simulink model "Heli_Simulation_VR1"  (R2024b)
settings: Solver=FixedStepAuto  StartTime=0.0  StopTime=50  RelTol=1e-3  EnableMultiTasking=on
values from neighbouring files (symbols this model uses):
  D2R = pi/180.0    (= 0.0174532925199)    [Heli_Setup.m]
  ELEV_SLF = 24.25    [Heli_Setup.m]
  ELEV_START = -24.25    [Heli_Setup.m]
  Kd = 128    [Heli_Setup.m]
  Kdt = 1.38e3    (= 1380)    [Heli_Setup.m]
  Ki = 63.5    [Heli_Setup.m]
  Kit = 43.4    [Heli_Setup.m]
  Kp = 84.1    [Heli_Setup.m]
  Kpt = 448    [Heli_Setup.m]
  R2D = 180/pi    (= 57.2957795131)    [Heli_Setup.m]
  VSUM_MAX = 36    [Heli_Setup.m]
undefined symbols (not defined in the file or in its folder): YAW_SP, YAW_START
libraries: vrlib x7, cstblocks x2
Description:
  | Simulink(R) 3D Animation(TM) - Tutorial #3
  | 
  | Tutorial model to be used for 3D World Editor authoring example in the documentation.
  | After creating the virtual world according to the instructions in the documentation, include the VR block
  | in the model and connect B1, B2 coordinates and S scaling to corresponding nodes in
  | the virtual world.
settings Model: Creator=Danek  LastModifiedBy=bryankikuta
settings SolverCC: ConcurrentTasks=on  AlgebraicLoopSolver=TrustRegion  AutoInsertRateTranBlk=on  InsertRTBMode=Never (minimum delay)
settings DataIOCC: LimitDataPoints=on  SaveFormat=StructureWithTime  SignalLoggingSaveFormat=ModelDataLogs  SaveOutput=off  SaveTime=off  ReturnWorkspaceOutputs=off  SignalLoggingName=logsOut
settings OptimizationCC: BlockReduction=off  BooleanDataType=off  DefaultParameterBehavior=Inlined  OptimizeBlockIOStorage=off  BufferReuse=off  GlobalBufferReuse=off  ExpressionFolding=off  PassReuseOutputArgsThreshold=0  ExpressionDepthLimit=2147483647  LocalBlockOutputs=off  InitFltsAndDblsToZero=on
settings DebuggingCC: UnderspecifiedInitializationDetection=Classic  MergeDetectMultiDrivingBlocksExec=none  CheckExecutionContextPreStartOutputMsg=on  SignalResolutionControl=TryResolveAllWithWarning  ParameterTunabilityLossMsg=error  FcnCallInpInsideContextMsg=warning  UnconnectedInputMsg=warning  UnconnectedOutputMsg=warning  UnconnectedLineMsg=warning  StateNameClashWarn=warning  SFUnexpectedBacktrackingDiag=warning  SFNoUnconditionalDefaultTransitionDiag=warning  SFExecutionAtInitializationDiag=none  ArithmeticOperatorsInVariantConditions=warning
settings HardwareCC: TargetBitPerLong=64  TargetBitPerPointer=64  TargetBitPerSizeT=64  TargetBitPerPtrDiffT=64  TargetLongLongMode=on  TargetIntDivRoundTo=Zero  TargetEndianess=LittleEndian  TargetWordSize=64  TargetHWDeviceType=MATLAB Host
settings ModelReferenceCC: UpdateModelReferenceTargets=IfOutOfDate  EnableRefExpFcnMdlSchedulingChecks=on  PropagateSignalLabelsOutOfModel=off
settings SFSimCC: SimUseLocalCustomCode=off  MATLABDynamicMemAlloc=off  CustomCodeUndefinedFunction=UseInterfaceOnly
settings RTWCC: GenerateReport=on  RTWUseLocalCustomCode=off  LaunchReport=on  RTWCompilerOptimization=on  GPUComputeCapability=3.5
settings CodeAppCC: ForceParamTrailComments=on  MaxIdLength=95  OperatorAnnotations=on  StateflowObjectComments=on  MATLABSourceComments=on
settings GRTTargetCC: TargetLangStandard=C89/C90 (ANSI)
settings ConfigComp: CovMetricSettings=d  CovSaveCumulativeToWorkspaceVar=on  CovSaveSingleToWorkspaceVar=on  CovExternalEMLEnable=off

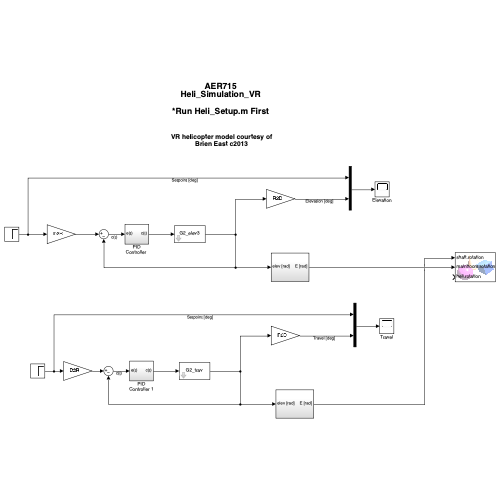
[thumbnail: Simulink's stored preview of the top-level diagram]
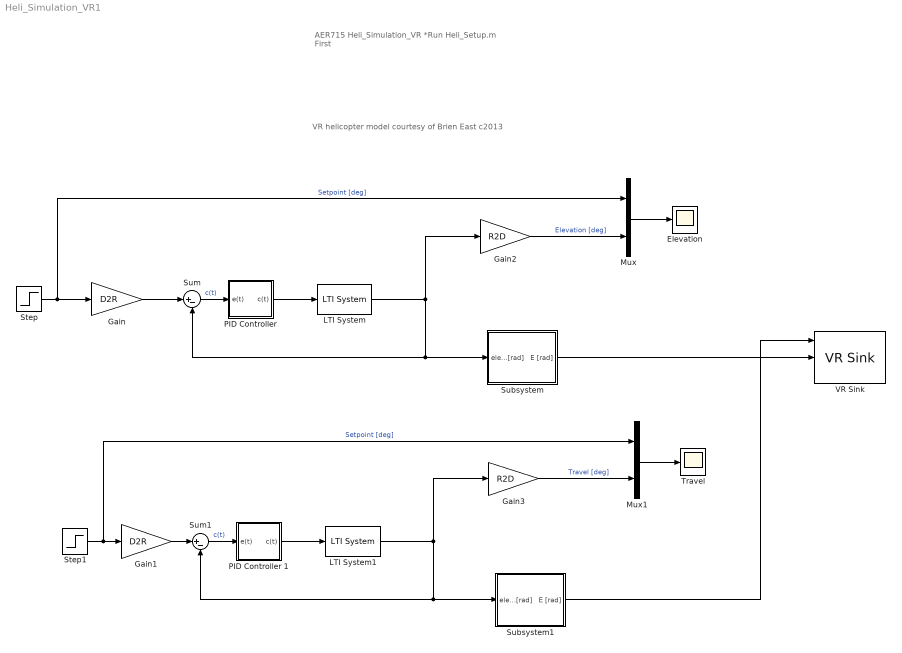
== system Heli_Simulation_VR1 ==
  note: AER715
      | Heli_Simulation_VR
      |
      | *Run Heli_Setup.m First
  note: VR helicopter model courtesy of
      | Brien East c2013
  " PID Controller " : Subsystem
  " PID Controller 1" : Subsystem
  Elevation : Scope
  Gain : Gain  Gain=D2R
  Gain1 : Gain  Gain=D2R
  Gain2 : Gain  Gain=R2D
  Gain3 : Gain  Gain=R2D
  LTI System : cstblocks/LTI System  sys=G2_elev3  IC=[]  PadeOrder=0
  LTI System1 : cstblocks/LTI System  sys=G2_trav  IC=[]  PadeOrder=0
  Mux : Mux  Inputs=2
  Mux1 : Mux  Inputs=2
  Step : Step  Before=ELEV_START  After=ELEV_SLF  SampleTime=0.1
  Step1 : Step  Before=YAW_START  After=YAW_SP  SampleTime=0.1
  Subsystem : Subsystem
  Subsystem1 : Subsystem
  Sum : Sum  Inputs=|+-
  Sum1 : Sum  Inputs=|+-
  Travel : Scope
  VR Sink : vrlib/VR Sink  InstantiateOnLoad=on  SampleTime=-1  ViewEnable=on  RemoteChange=off  RemoteView=off  FieldsWritten=shaft.rotation.4.1.1.double#mainboom.rotation.4.1.1.double#heli.rotation.4.1.1.double  WorldFileName=heliMain.wrl  AutoView=on  VideoDimensions=[]  AllowVariableSize=off
  wires:
  LTI System/1 -> Gain2/1, Sum/2, Subsystem/1(elev [rad])
  Subsystem/1(E [rad]) -> VR Sink/2
  Gain/1 -> Sum/1
  Sum/1 -> " PID Controller "/1(e(t))  "c(t)"
  " PID Controller "/1(c(t)) -> LTI System/1
  Gain2/1 -> Mux/2  "Elevation [deg]"
  Mux/1 -> Elevation/1
  Step/1 -> Gain/1, Mux/1  "Setpoint [deg]"
  LTI System1/1 -> Gain3/1, Sum1/2, Subsystem1/1(elev [rad])
  Subsystem1/1(E [rad]) -> VR Sink/1
  Gain1/1 -> Sum1/1
  Sum1/1 -> " PID Controller 1"/1(e(t))  "c(t)"
  " PID Controller 1"/1(c(t)) -> LTI System1/1
  Gain3/1 -> Mux1/2  "Travel [deg]"
  Mux1/1 -> Travel/1
  Step1/1 -> Gain1/1, Mux1/1  "Setpoint [deg]"

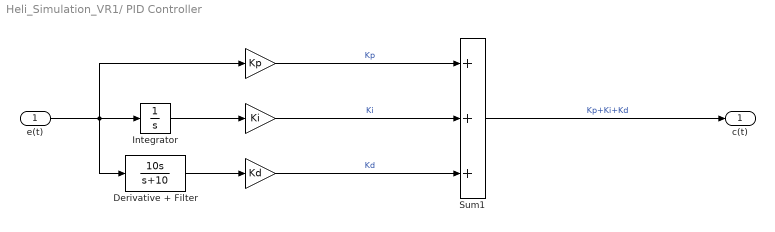
== system Heli_Simulation_VR1/ PID Controller  ==
  e(t) : Inport
  " " : Gain  Gain=Kp
  "  " : Gain  Gain=Ki
  "   " : Gain  Gain=Kd
  Derivative + Filter : TransferFcn  Numerator=[10 0]  Denominator=[1 10]
  Integrator : Integrator  UpperSaturationLimit=30  LowerSaturationLimit=-30
  Sum1 : Sum  Inputs=+++
  c(t) : Outport
  wires:
  " "/1 -> Sum1/1  "Kp"
  Sum1/1 -> c(t)/1  "Kp+Ki+Kd"
  "  "/1 -> Sum1/2  "Ki"
  "   "/1 -> Sum1/3  "Kd"
  Derivative + Filter/1 -> "   "/1
  Integrator/1 -> "  "/1
  e(t)/1 -> Integrator/1, Derivative + Filter/1, " "/1

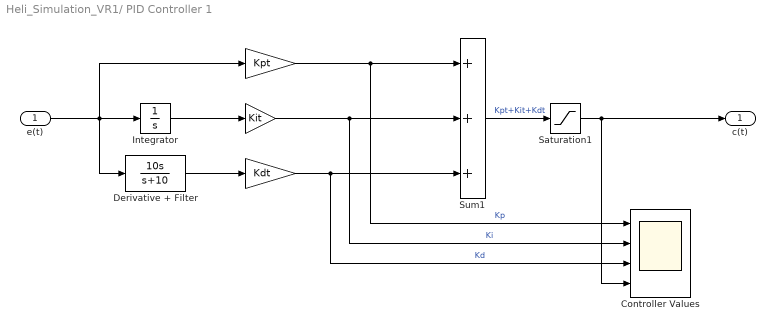
== system Heli_Simulation_VR1/ PID Controller 1 ==
  e(t) : Inport
  " " : Gain  Gain=Kpt
  "  " : Gain  Gain=Kit
  "   " : Gain  Gain=Kdt
  Controller Values : Scope  NumInputPorts=4
  Derivative + Filter : TransferFcn  Numerator=[10 0]  Denominator=[1 10]
  Integrator : Integrator  UpperSaturationLimit=30  LowerSaturationLimit=-30
  Saturation1 : Saturate  UpperLimit=VSUM_MAX  LowerLimit=-VSUM_MAX
  Sum1 : Sum  Inputs=+++
  c(t) : Outport
  wires:
  " "/1 -> Sum1/1, Controller Values/1  "Kp"
  "  "/1 -> Sum1/2, Controller Values/2  "Ki"
  "   "/1 -> Sum1/3, Controller Values/3  "Kd"
  Derivative + Filter/1 -> "   "/1
  Integrator/1 -> "  "/1
  e(t)/1 -> Integrator/1, Derivative + Filter/1, " "/1
  Sum1/1 -> Saturation1/1  "Kpt+Kit+Kdt"
  Saturation1/1 -> Controller Values/4, c(t)/1

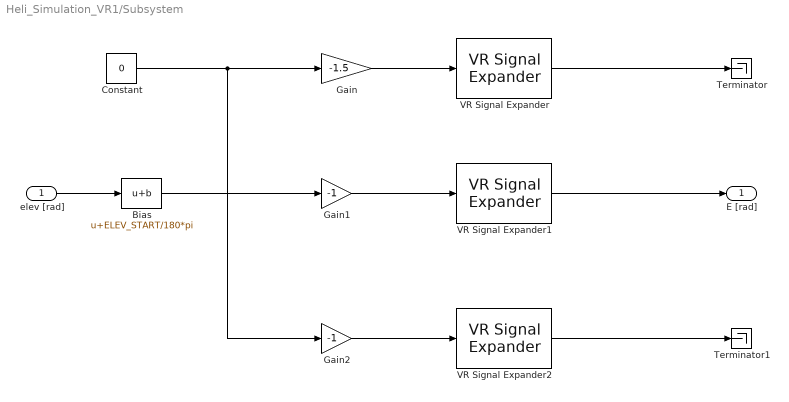
== system Heli_Simulation_VR1/Subsystem ==
  elev [rad] : Inport
  Bias : Bias  Bias=ELEV_START/180*pi  SaturateOnIntegerOverflow=off
  Constant : Constant  Value=0
  Gain : Gain  Gain=-1.5
  Gain1 : Gain  Gain=-1
  Gain2 : Gain  Gain=-1
  Terminator : Terminator
  Terminator1 : Terminator
  VR Signal Expander : vrlib/VR Signal Expander  outwidth=4  outidx=4
  VR Signal Expander1 : vrlib/VR Signal Expander  outwidth=4  outidx=4
  VR Signal Expander2 : vrlib/VR Signal Expander  outwidth=4  outidx=4
  E [rad] : Outport
  wires:
  elev [rad]/1 -> Bias/1
  Gain/1 -> VR Signal Expander/1
  Constant/1 -> Gain2/1, Gain/1
  VR Signal Expander1/1 -> E [rad]/1
  Gain1/1 -> VR Signal Expander1/1
  Gain2/1 -> VR Signal Expander2/1
  Bias/1 -> Gain1/1
  VR Signal Expander2/1 -> Terminator1/1
  VR Signal Expander/1 -> Terminator/1

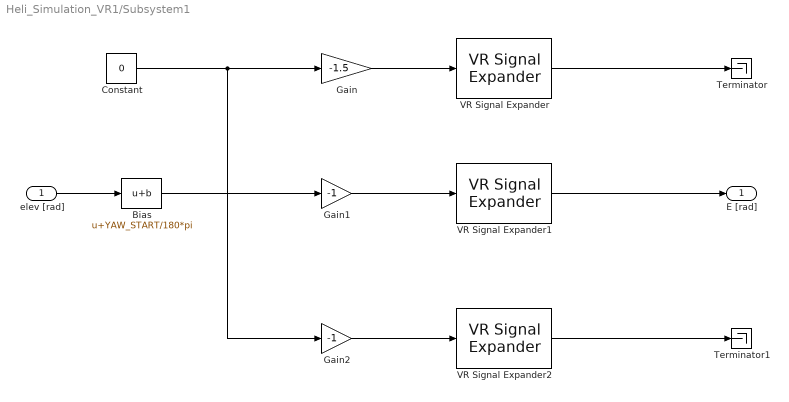
== system Heli_Simulation_VR1/Subsystem1 ==
  elev [rad] : Inport
  Bias : Bias  Bias=YAW_START/180*pi  SaturateOnIntegerOverflow=off
  Constant : Constant  Value=0
  Gain : Gain  Gain=-1.5
  Gain1 : Gain  Gain=-1
  Gain2 : Gain  Gain=-1
  Terminator : Terminator
  Terminator1 : Terminator
  VR Signal Expander : vrlib/VR Signal Expander  outwidth=4  outidx=4
  VR Signal Expander1 : vrlib/VR Signal Expander  outwidth=4  outidx=4
  VR Signal Expander2 : vrlib/VR Signal Expander  outwidth=4  outidx=4
  E [rad] : Outport
  wires:
  elev [rad]/1 -> Bias/1
  Gain/1 -> VR Signal Expander/1
  Constant/1 -> Gain2/1, Gain/1
  Gain1/1 -> VR Signal Expander1/1
  Gain2/1 -> VR Signal Expander2/1
  Bias/1 -> Gain1/1
  VR Signal Expander2/1 -> Terminator1/1
  VR Signal Expander/1 -> Terminator/1
  VR Signal Expander1/1 -> E [rad]/1
